simulink model "Ej2"  (R2023a)
settings: Solver=VariableStepAuto  StartTime=0.0  StopTime=20  RelTol=1e-3
undefined symbols (not defined in the file or in its folder): magnitude
settings Model: Creator=santi  LastModifiedBy=santi

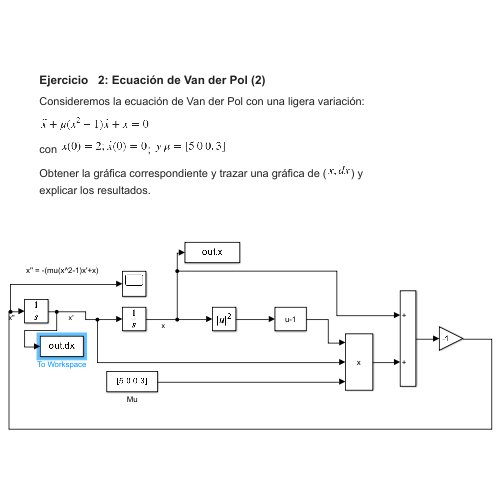
[thumbnail: Simulink's stored preview of the top-level diagram]
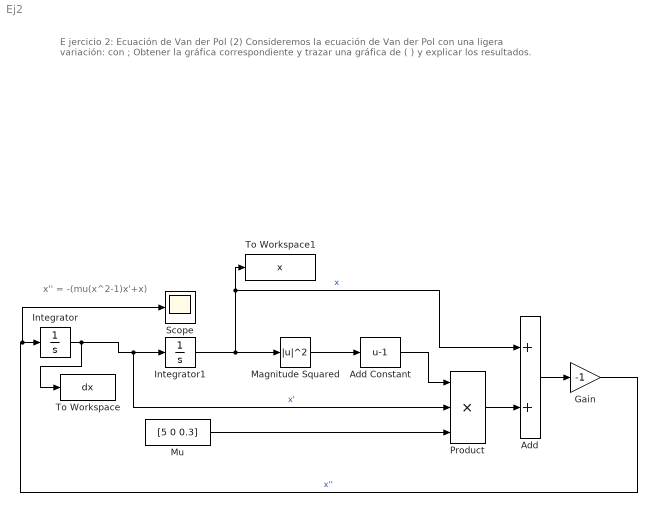
== system Ej2 ==
  note: x'' = -(mu(x^2-1)x'+x)
  note: E jercicio 2: Ecuación de Van der Pol (2)
      | Consideremos la ecuación de Van der Pol con una ligera variación:
      |
      | con ;
      | Obtener la gráfica correspondiente y trazar una gráfica de ( ) y explicar los resultados.
  Add : Sum
  Add Constant : Bias  Bias=-1  SaturateOnIntegerOverflow=off
  Gain : Gain  Gain=-1
  Integrator : Integrator
  Integrator1 : Integrator  InitialCondition=2
  Magnitude Squared : Math  Operator=magnitude^2
  Mu : Constant  Value=[5 0 0.3]
  Product : Product  Inputs=3
  Scope : Scope
  To Workspace : ToWorkspace  VariableName=dx  SampleTime=-1
  To Workspace1 : ToWorkspace  VariableName=x  SampleTime=-1
  wires:
  Gain/1 -> Scope/1, Integrator/1  "x''"
  Integrator/1 -> To Workspace/1, Product/2, Integrator1/1  "x'"
  Integrator1/1 -> Magnitude Squared/1, To Workspace1/1, Add/1  "x"
  Magnitude Squared/1 -> Add Constant/1
  Add Constant/1 -> Product/1
  Mu/1 -> Product/3
  Product/1 -> Add/2
  Add/1 -> Gain/1
